simulink model "Example"  (R2017b)
settings: Solver=FixedStepAuto  StartTime=0.0  StopTime=inf  FixedStep=0.1  RelTol=1e-3  EnableMultiTasking=on
libraries: OBD2_SocketCan_Library x1
settings Model: SimulationMode=external  Creator=Murml  LastModifiedBy=Murml
settings SolverCC: PositivePriorityOrder=on
settings OptimizationCC: PassReuseOutputArgsThreshold=0  MaxStackSize=64
settings DebuggingCC: ParameterTunabilityLossMsg=error
settings HardwareCC: ProdBitPerPointer=32  ProdBitPerSizeT=32  ProdBitPerPtrDiffT=32  ProdLargestAtomicInteger=Long  ProdLargestAtomicFloat=Double  ProdWordSize=32  ProdHWDeviceType=ARM Compatible->ARM Cortex  UseEmbeddedCoderFeatures=off
settings SFSimCC: MATLABDynamicMemAlloc=off
settings RTWCC: SystemTargetFile=ert.tlc  HardwareBoard=Raspberry Pi  TemplateMakefile=ert_default_tmf  Toolchain=GNU GCC Raspberry Pi
settings CodeAppCC: ForceParamTrailComments=on  OperatorAnnotations=on
settings ERTTargetCC: ERTCustomFileBanners=off  SupportContinuousTime=on  SupportNonInlinedSFcns=on  RemoveResetFunc=off  SupportVariableSizeSignals=on  ModelStepFunctionPrototypeControlCompliant=off

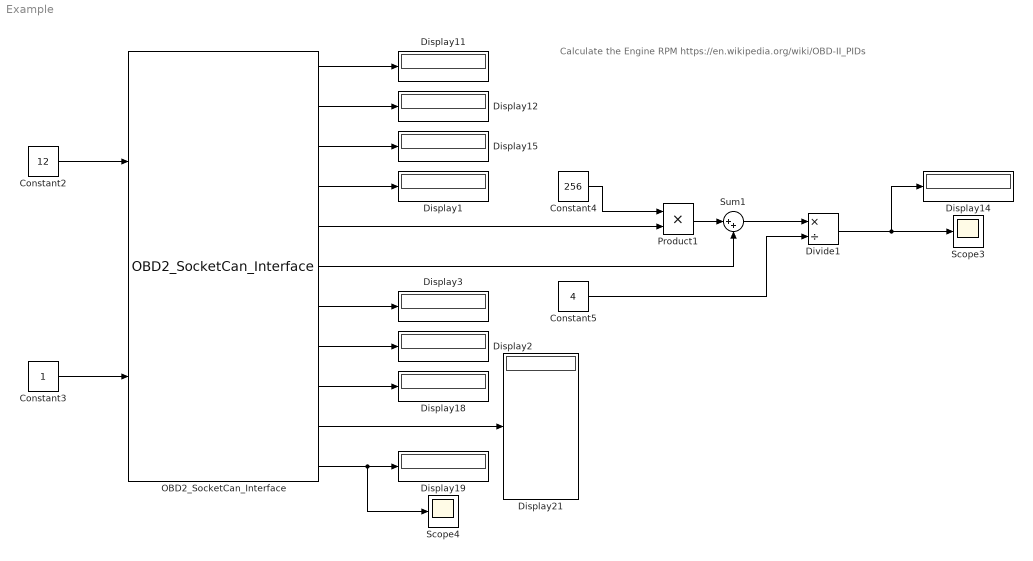
== system Example ==
  note: Calculate the Engine RPM
      | https://en.wikipedia.org/wiki/OBD-II_PIDs
  Constant2 : Constant  Value=12  OutDataTypeStr=uint8  SampleTime=-1
  Constant3 : Constant  OutDataTypeStr=uint8  SampleTime=-1
  Constant4 : Constant  Value=256  SampleTime=-1
  Constant5 : Constant  Value=4  SampleTime=-1
  Display{1..3,11..12,14..15,18..19,21} (10 alike) : Display
      Display11 settings: Format=hex (Stored Integer)
  Divide1 : Product  Inputs=*/
  OBD2_SocketCan_Interface : OBD2_SocketCan_Library/OBD2_SocketCan_Interface  sampleTime=0.1
      settings: SourceProductName=OBD2 SocketCan Interface
  Product1 : Product
  Scope3 : Scope
  Scope4 : Scope
  Sum1 : Sum  Inputs=|++
  wires:
  Constant3/1 -> OBD2_SocketCan_Interface/2
  Constant2/1 -> OBD2_SocketCan_Interface/1
  OBD2_SocketCan_Interface/3 -> Display15/1
  Divide1/1 -> Display14/1, Scope3/1
  OBD2_SocketCan_Interface/5 -> Product1/2
  OBD2_SocketCan_Interface/9 -> Display18/1
  Constant5/1 -> Divide1/2
  OBD2_SocketCan_Interface/1 -> Display11/1
  OBD2_SocketCan_Interface/2 -> Display12/1
  OBD2_SocketCan_Interface/6 -> Sum1/2
  Sum1/1 -> Divide1/1
  Product1/1 -> Sum1/1
  Constant4/1 -> Product1/1
  OBD2_SocketCan_Interface/4 -> Display1/1
  OBD2_SocketCan_Interface/7 -> Display3/1
  OBD2_SocketCan_Interface/8 -> Display2/1
  OBD2_SocketCan_Interface/11 -> Scope4/1, Display19/1
  OBD2_SocketCan_Interface/10 -> Display21/1
